simulink model "hvdc_gfm_bess"  (R2024a)
settings: Solver=ode23tb  StartTime=0.0  StopTime=10  MaxStep=2e-4  RelTol=1e-7  AbsTol=1e-9
settings Model: Creator=Birane  LastModifiedBy=Birane

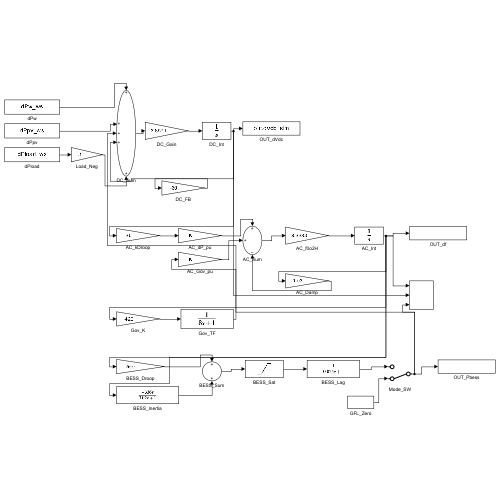
[thumbnail: Simulink's stored preview of the top-level diagram]
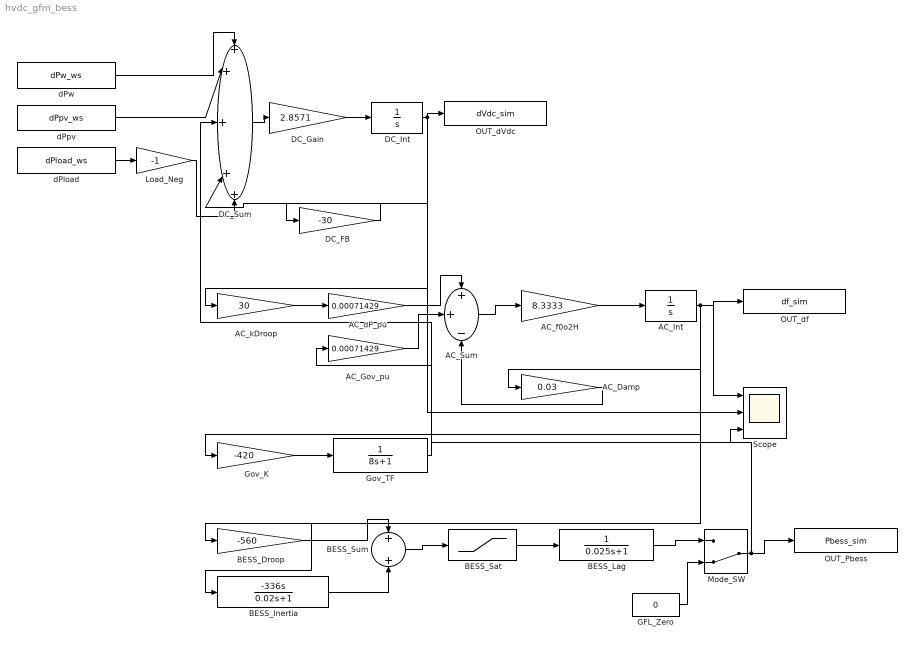
== system hvdc_gfm_bess ==
  AC_Damp : Gain  Gain=0.03
  AC_Gov_pu : Gain  Gain=0.00071429
  AC_Int : Integrator
  AC_Sum : Sum  Inputs=++-
  AC_dP_pu : Gain  Gain=0.00071429
  AC_f0o2H : Gain  Gain=8.3333
  AC_kDroop : Gain  Gain=30
  BESS_Droop : Gain  Gain=-560
  BESS_Inertia : TransferFcn  Numerator=[-336 0]  Denominator=[0.02 1]
  BESS_Lag : TransferFcn  Denominator=[0.025 1]
  BESS_Sat : Saturate  UpperLimit=200  LowerLimit=-50
  BESS_Sum : Sum
  DC_FB : Gain  Gain=-30
  DC_Gain : Gain  Gain=2.8571
  DC_Int : Integrator
  DC_Sum : Sum  Inputs=+++++
  GFL_Zero : Constant  Value=0
  Gov_K : Gain  Gain=-420
  Gov_TF : TransferFcn  Denominator=[8 1]
  Load_Neg : Gain  Gain=-1
  Mode_SW : ManualSwitch  CurrentSetting=0
  OUT_Pbess : ToWorkspace  VariableName=Pbess_sim  SampleTime=-1
  OUT_dVdc : ToWorkspace  VariableName=dVdc_sim  SampleTime=-1
  OUT_df : ToWorkspace  VariableName=df_sim  SampleTime=-1
  Scope : Scope  NumInputPorts=3
  dPload : FromWorkspace  VariableName=dPload_ws
  dPpv : FromWorkspace  VariableName=dPpv_ws
  dPw : FromWorkspace  VariableName=dPw_ws
  wires:
  dPw/1 -> DC_Sum/1
  dPpv/1 -> DC_Sum/2
  DC_FB/1 -> DC_Sum/4
  dPload/1 -> Load_Neg/1
  Load_Neg/1 -> DC_Sum/5
  DC_Sum/1 -> DC_Gain/1
  DC_Gain/1 -> DC_Int/1
  DC_Int/1 -> OUT_dVdc/1, DC_FB/1, AC_kDroop/1, Scope/2
  AC_kDroop/1 -> AC_dP_pu/1
  AC_dP_pu/1 -> AC_Sum/1
  AC_Sum/1 -> AC_f0o2H/1
  AC_f0o2H/1 -> AC_Int/1
  AC_Int/1 -> OUT_df/1, Scope/1, AC_Damp/1, Gov_K/1, BESS_Droop/1, BESS_Inertia/1
  AC_Damp/1 -> AC_Sum/3
  Gov_K/1 -> Gov_TF/1
  Gov_TF/1 -> AC_Gov_pu/1
  AC_Gov_pu/1 -> AC_Sum/2
  BESS_Droop/1 -> BESS_Sum/1
  BESS_Inertia/1 -> BESS_Sum/2
  BESS_Sum/1 -> BESS_Sat/1
  BESS_Sat/1 -> BESS_Lag/1
  BESS_Lag/1 -> Mode_SW/1
  GFL_Zero/1 -> Mode_SW/2
  Mode_SW/1 -> DC_Sum/3, OUT_Pbess/1, Scope/3
